simulink model "Sub2_2023"  (R2023b)
settings: Solver=FixedStepDiscrete  StartTime=0.0  StopTime=4.5  FixedStep=7.5e-05  RelTol=1e-3  EnableMultiTasking=on
undefined symbols (not defined in the file or in its folder): D1, D11, Delta
libraries: spsSeriesRLCBranchLib x41, spsLoadFlowBusLib x29, spsDistributedParametersLineLib x19, spsThreePhaseSeriesRLCLoadLib x15, spsThreePhaseTransformerTwoWindingsLib x13, spsThreePhaseParallelRLCLoadLib x11, spsThreePhaseVIMeasurementLib x11, spsSynchronousMachinepuStandardLib x7, spsExcitationSystemLib x7, spsHydraulicTurbineandGovernorLib x7, spsGenericPowerSystemStabilizerLib x7, spsMultiBandPowerSystemStabilizerLib x7
(part 1 of 5)
settings Model: Creator=The MathWorks, Inc.  LastModifiedBy=dilu2
settings SolverCC: AlgebraicLoopSolver=TrustRegion
settings DataIOCC: SaveFormat=StructureWithTime  SaveOutput=off  SignalLogging=off  DSMLogging=off  SaveTime=off  ReturnWorkspaceOutputs=off
settings OptimizationCC: ExpressionDepthLimit=2147483647  LifeSpan=inf
settings DebuggingCC: UnderspecifiedInitializationDetection=Classic  MergeDetectMultiDrivingBlocksExec=none  SolverPrmCheckMsg=warning  FcnCallInpInsideContextMsg=warning  UnconnectedInputMsg=warning  UnconnectedOutputMsg=warning  UnconnectedLineMsg=warning  StateNameClashWarn=warning  SFUnexpectedBacktrackingDiag=warning  SFNoUnconditionalDefaultTransitionDiag=warning  SFExecutionAtInitializationDiag=none  ArithmeticOperatorsInVariantConditions=warning
settings HardwareCC: ProdBitPerPointer=32  ProdBitPerSizeT=32  ProdBitPerPtrDiffT=32  ProdLargestAtomicFloat=None  ProdIntDivRoundTo=Undefined  ProdEndianess=Unspecified  ProdWordSize=32  ProdHWDeviceType=32-bit Generic
settings ModelReferenceCC: EnableRefExpFcnMdlSchedulingChecks=on  PropagateSignalLabelsOutOfModel=off
settings SFSimCC: SimUseLocalCustomCode=off  CustomCodeUndefinedFunction=UseInterfaceOnly
settings RTWCC: RTWUseLocalCustomCode=off
settings CodeAppCC: StateflowObjectComments=on
settings GRTTargetCC: TargetLangStandard=C89/C90 (ANSI)  CombineOutputUpdateFcns=off  GRTInterface=on
settings ConfigComp: CovMetricSettings=dw  CovSaveCumulativeToWorkspaceVar=on  CovSaveSingleToWorkspaceVar=on  CovExternalEMLEnable=off  CovSFcnEnable=off
settings SimscapeCC: SimscapeNormalizeSystem=off

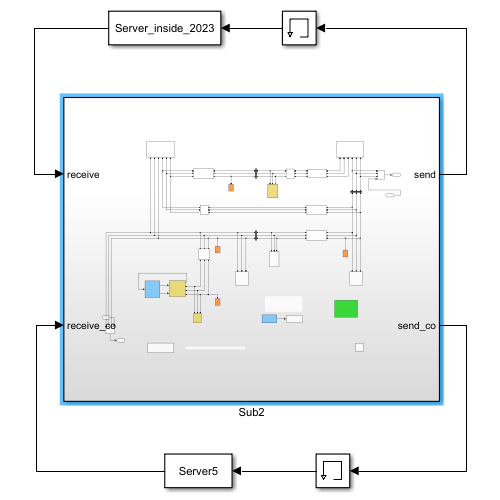
[thumbnail: Simulink's stored preview of the top-level diagram]
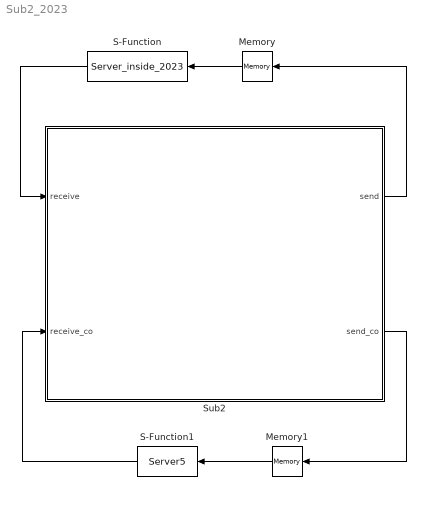
== system Sub2_2023 ==
  Memory : Memory
  Memory1 : Memory
  S-Function : S-Function  FunctionName=Server_inside_2023  SFunctionDeploymentMode=off  EnableBusSupport=off
  S-Function1 : S-Function  FunctionName=Server5  SFunctionDeploymentMode=off  EnableBusSupport=off
  Sub2 : Subsystem
  wires:
  Memory/1 -> S-Function/1
  Sub2/1(send) -> Memory/1
  S-Function/1 -> Sub2/1(receive)
  Memory1/1 -> S-Function1/1
  Sub2/2(send_co) -> Memory1/1
  S-Function1/1 -> Sub2/2(receive_co)

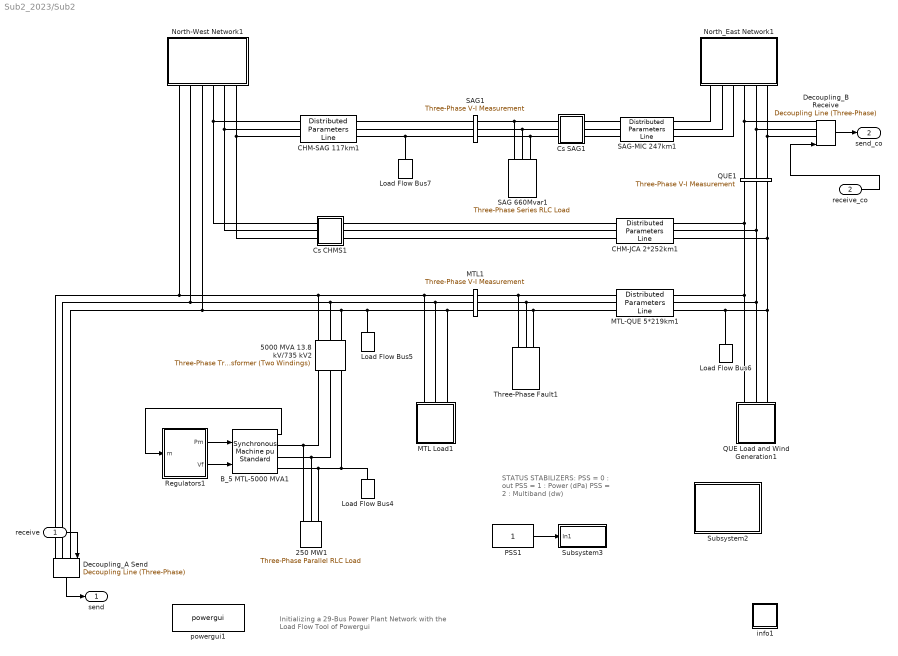
== system Sub2_2023/Sub2 ==
  note: STATUS STABILIZERS:
      | PSS = 0 :  out
      | PSS = 1 :  Power (dPa)
      | PSS = 2 :  Multiband (dw)
  note: Initializing a 29-Bus Power Plant Network with the Load Flow Tool of Powergui
  receive : Inport
  receive_co : Inport  Port=2
  250 MW1 : spsThreePhaseParallelRLCLoadLib/Three-Phase Parallel RLC Load  LConnTagsString=A|B|C  Configuration=Y (grounded)  NominalVoltage=(13800)*1  Vabc=[1e3 1e3 1e3]  Vabcp=[1e3 1e3 1e3]  NominalFrequency=60  UnbalancedPower=off  ActivePower=250000000  InductivePower=0  CapacitivePower=0  Pabc=[10e3 9e3 11e3]  QLabc=[100 90 110]  QCabc=[100 90 110]  Pabcp=[10e3 9e3 11e3]  QLabcp=[100 90 110]  QCabcp=[100 90 110]  Measurements=None  LoadType=constant PQ
  5000 MVA 13.8 kV/735 kV2 : spsThreePhaseTransformerTwoWindingsLib/Three-Phase Transformer (Two Windings)  Winding1Connection=Delta (D1)  Winding2Connection=Yg  CoreType=Three single-phase transformers  SetSaturation=off  Hysteresis=off  DataFile='basic_model'  SetInitialFlux=off  Measurements=None  UNITS=pu  NominalPower=[ 5000e6 60 ]  Winding1="[ 13.8e3 0.002  0.0]"  Winding2=[ 735e3 0.002 0.12]  Rm=500  Lm=500  L0=0.5  Saturation="[ 0,0  ;  0.005,1.2  ;  1.0,1.4 ]"  InitialFluxes=[ 0.8 , -0.8 , 0.7 ]  BreakLoop=off  DiscreteSolver=Trapezoidal iterative  DataType=off  TransfoNumber=0
  B_5 MTL-5000 MVA1 : spsSynchronousMachinepuStandardLib/Synchronous Machine pu Standard  PresetModel=No  MechanicalLoad=Mechanical power Pm  ShowDetailedParameters=on  RotorType=Salient-pole  Units=per unit standard parameters  MeasurementBus=off  NominalParameters="[5000E6  13800   60 ]"  Reactances1=[ 31 32 33 34 35 36 37 ]  Reactances2=[ 1.305, 0.296, 0.252, 0.474, 0.243, 0.18 ]  dAxisTimeConstants=Short-circuit  qAxisTimeConstants=Open-circuit  TimeConstants1=[]  TimeConstants2=[]  TimeConstants3=[]  TimeConstants4=[]  TimeConstants5=[ 1.01, 0.053, 0.1 ]  TimeConstants6=[]  TimeConstants7=[]  TimeConstants8=[]  StatorResistance=2.8544e-3  Mechanical="[ 3.7 0  32]"  PolePairs=32  InitialConditions=[0 -113.876 0.904539 0.904539 0.904539 -42.1129 -162.113 77.8871 1.28555]  SetSaturation=off  Saturation=[0.6404,0.7127,0.8441,0.9214,0.9956,1.082,1.19,1.316,1.457;0.7,0.7698,0.8872,0.9466,0.9969,1.046,1.1,1.151,1.201]  LoadFlowParameters=[1 4000000000 0 0 0]  TsPowergui=0  TsBlock=-1  IterativeModel=Trapezoidal non iterative  IterativeDiscreteModel=Trapezoidal non iterative  BusType=PV  Pref=4500000000  Qref=0  Qmin=-Inf  Qmax=Inf  PLF=0  QLF=0
  CHM-JCA 2*252km1 : spsDistributedParametersLineLib/Distributed Parameters Line  Phases=3  Length=252  Frequency=60  Resistance="[0.01273  0.3864]/2"  Inductance="[0.9337e-3  4.1264e-3]/2"  Capacitance=[12.74e-9 7.751e-9]*2  x1=[-0.0015 2.03650540175105e-08 15714.2625948623 -742648.807936856;-0.001425 2.03802417175712e-08 36703.0761534736 -741907.711972361;-0.00135 2.03791377642309e-08 57662.5498345837 -740573.546334484;-0.001275 2.03617430399732e-08 78575.9289556225 -738647.377534823;-0.0012 2.03280714498745e-08 99426.4956813062 -736130.745323245;-0.001125 2.02781499104887e-08 120197.582387619 -733025.661457033;-0.00105 2.02120183283305e-08 140872.584985655 -729334.608092721;-0.000975 2.01297295679749e-08 161434.976194677 -725060.535801893;-0.0009 2.00313494097978e-08 181868.318753767 -720206.861212544;-0.000825 1.99169564973925e-08 202156.278561524 -714777.464277876;-0.00075 1.97866422747028e-08 222282.637733293 -708776.685174726;-0.000675 1.96405109129245e-08 242231.307565497 -702209.320834094;-0.0006 1.94786792272323e-08 261986.341396696 -695080.621106551;-0.000525 1.93012765833996e-08 281531.947355108 -687396.284565585;-0.00045 1.91084447943856e-08 300852.500982388 -679162.453952253;-0.000375 1.8900338006972e-08 319932.55772358 -670385.711264765;-0.0003 1.86771225785405e-08 338756.86527326 -661073.072496938;-0.000225 1.84389769440892e-08 357310.375767994 -651231.982029715;-0.00015 1.81860914735947e-08 375578.257815372 -640870.306680239;-7.5e-05 1.79186683198327e-08 393545.908349992 -629996.329413249]  x2=[-0.0015 1.37456476437626e-08 -209700.603633318 -700128.672635041;-0.001425 1.37143974011628e-08 -189823.746323575 -705777.196573853;-0.00135 1.36721840791177e-08 -169795.146815422 -710861.533020477;-0.001275 1.36190414223113e-08 -149630.815664857 -715377.617634151;-0.0012 1.35550119121701e-08 -129346.871929678 -719321.840325932;-0.001125 1.34801467329051e-08 -108959.530284152 -722691.048144551;-0.00105 1.33945057305949e-08 -88485.088057253 -725482.547796826;-0.000975 1.32981573653464e-08 -67939.9122048287 -727694.107800648;-0.0009 1.31911786565688e-08 -47340.4262261034 -729323.960268787;-0.000825 1.30736551214049e-08 -26703.0970349858 -730370.802322118;-0.00075 1.29456807063705e-08 -6044.42179666949 -730833.797131121;-0.000675 1.28073577122551e-08 14619.0852599484 -730712.574584829;-0.0006 1.26587967123436e-08 35270.9060434889 -730007.231586691;-0.000525 1.25001164640264e-08 55894.5318044012 -728718.331977109;-0.00045 1.2331443813866e-08 76473.4763318042 -726846.906082708;-0.000375 1.21529135961982e-08 96991.2891323108 -724394.449892715;-0.0003 1.19646685253474e-08 117431.568580302 -721362.923863085;-0.000225 1.1766859081543e-08 137777.975029133 -717754.751349341;-0.00015 1.15596433906279e-08 158014.243872799 -713572.816669385;-7.5e-05 1.13431870976547e-08 178124.198547612 -708820.462797813]  x3=[-0.0015 5.03591321245588e-11 0.894999888084755 -284.908126311335;-0.001425 4.98693784000735e-11 8.94952227197466 -284.768519996507;-0.00135 4.93397598575223e-11 16.9968905446926 -284.401274083898;-0.001275 4.87706998658647e-11 25.0306717631703 -283.806682144272;-0.0012 4.8162653322951e-11 33.0444438456226 -282.985219485328;-0.001125 4.75161062918843e-11 41.0318007052617 -281.937542771746;-0.00105 4.68315756124686e-11 48.9863573712246 -280.664489500261;-0.000975 4.61096084880555e-11 56.9017550926213 -279.167077330181;-0.0009 4.53507820481176e-11 64.7716664216231 -277.446503269882;-0.000825 4.45557028869008e-11 72.5898002715271 -275.504142719944;-0.00075 4.37250065785213e-11 80.3499069457553 -273.341548373669;-0.000675 4.28593571688979e-11 88.0457831337658 -270.960448975891;-0.0006 4.19594466449239e-11 95.6712768698848 -268.362747941035;-0.000525 4.1025994381303e-11 103.220292451094 -265.550521831563;-0.00045 4.00597465654924e-11 110.686795309841 -262.526018697998;-0.000375 3.9061475601212e-11 118.064816837982 -259.291656281869;-0.0003 3.80319794909967e-11 125.348459157995 -255.850020083003;-0.000225 3.69720811982851e-11 132.531899837652 -252.20386129272;-0.00015 3.58826279895553e-11 139.609396544386 -248.356094594567;-7.5e-05 3.47644907570334e-11 146.575291635618 -244.309795834372]  x4=[-0.0015 3.52013720407501e-11 -3172.83341993516 -10043.3125795473;-0.001425 3.62675085587556e-11 -2887.63550825219 -10128.9965094932;-0.00135 3.73046533853308e-11 -2600.12926492622 -10206.5834746083;-0.001275 3.83119774427701e-11 -2310.54451804918 -10276.0114530598;-0.0012 3.92886754916345e-11 -2019.11275723693 -10337.224945184;-0.001125 4.02339667744478e-11 -1726.06694858001 -10390.1750178518;-0.00105 4.11470956398219e-11 -1431.6413484141 -10434.8193435853;-0.000975 4.20273321465133e-11 -1136.07131605911 -10471.1222343937;-0.0009 4.28739726469264e-11 -839.593125676545 -10499.0546703014;-0.000825 4.36863403495994e-11 -542.443777395516 -10518.5943225467;-0.00075 4.44637858602204e-11 -244.860807858507 -10529.7255714304;-0.000675 4.52056877007434e-11 52.9178996618098 -10532.4395188024;-0.0006 4.59114528061887e-11 350.654305422807 -10526.7339951749;-0.000525 4.65805169987294e-11 648.11040349724 -10512.6135614561;-0.00045 4.72123454386872e-11 945.048412031539 -10490.0895053046;-0.000375 4.78064330520745e-11 1241.23096332499 -10459.1798321063;-0.0003 4.83623049343428e-11 1536.42129357782 -10419.9092505811;-0.000225 4.88795167300147e-11 1830.3834321566 -10372.3091530309;-0.00015 4.93576549878944e-11 2122.88239022553 -10316.4175902454;-7.5e-05 4.97963374915741e-11 2413.68434859289 -10252.2792410848]  x5=0.00142516474882927  V1=ones(3,3)  V2=ones(3,3)  I1=ones(3,3)  I2=ones(3,3)  nHarmo=1  Measurements=None  Decoupling=on  VsMag0=[606505.937088319 606505.596193778 606505.952336297]  VrMag0=[596743.737336293 596743.911083344 596743.706580488]  VsAngle0=[3.61218308622256 -116.387796657594 123.612221103652]  VrAngle0=[-14.2738568821762 -134.273869923445 105.726122150017]  IsMag0=[234.023435046343 234.01262310882 234.010085806298]  IrMag0=[8650.90032066054 8650.9061903303 8650.91364627956]  IsAngle0=[2.58186505613148 -117.420380634198 122.583034804858]  IrAngle0=[-15.132183015214 -135.132103549665 104.867823050532]
      settings: AttributesFormatString=\n  LibrarySourceBlock=sps_lib/Power Grid Elements/Distributed Parameters Line
  CHM-SAG 117km1 : spsDistributedParametersLineLib/Distributed Parameters Line  Phases=3  Length=117  Frequency=60  Resistance="[0.01273  0.3864]"  Inductance="[0.9337e-3  4.1264e-3]"  Capacitance=[12.74e-9 7.751e-9]  x1=[-0.000675 1.88816449590376e-08 161384.253868467 -730188.013921256;-0.0006 1.87306893739895e-08 181962.578167366 -725333.731757354;-0.000525 1.85647607624449e-08 202395.444365398 -719899.628906264;-0.00045 1.83839917651972e-08 222666.51874196 -713890.04930666;-0.000375 1.81885268862169e-08 242759.59691035 -707309.796924525;-0.0003 1.79785223771376e-08 262658.616771318 -700164.13191293;-0.000225 1.77541461123506e-08 282347.671352849 -692458.766407155;-0.00015 1.75155774548089e-08 301811.021525966 -684199.859958489;-7.5e-05 1.72630071126472e-08 321033.108586338 -675394.01461038]  x2=[-0.000675 1.29951667225312e-08 211241.020698706 -709610.354234887;-0.0006 1.28653399577539e-08 231217.678579182 -703354.834381639;-0.000525 1.27252288370607e-08 251009.504585151 -696537.063435476;-0.00045 1.25749453631376e-08 270600.677433729 -689162.491418178;-0.000375 1.24146096702944e-08 289975.536241096 -681237.013449779;-0.0003 1.22443499284306e-08 309118.593041565 -672766.965036105;-0.000225 1.20643022405789e-08 328014.545168431 -663759.11700426;-0.00015 1.1874610534106e-08 346648.28748668 -654220.670090137;-7.5e-05 1.16754264456599e-08 365004.924467808 -644159.249182257]  x3=[-0.000675 1.4879769943779e-11 931.801693491408 -3923.77003572373;-0.0006 1.3949741165808e-11 1042.35686429537 -3895.8590867222;-0.000525 1.30085611781872e-11 1152.0787909706 -3864.83384757538;-0.00045 1.20569823457982e-11 1260.87976348774 -3830.71911938476;-0.000375 1.10957653461999e-11 1368.67280801404 -3793.54217294206;-0.0003 1.01256785615549e-11 1475.37175643902 -3753.33272692946;-0.000225 9.1474974643958e-12 1580.89131525584 -3710.12292416287;-0.00015 8.16200399772507e-12 1685.1471337437 -3663.94730589748;-7.5e-05 7.16998594994142e-12 1788.05587139646 -3614.84278421604]  x4=[-0.000675 2.80106439104315e-11 34.742941592912 -1477.3234716757;-0.0006 2.86931941198518e-11 76.4934319413538 -1475.75088744286;-0.000525 2.93528074289132e-11 118.182774610691 -1472.99861053035;-0.00045 2.99889565528289e-11 159.777643778261 -1469.06884106622;-0.000375 3.06011329637228e-11 201.244789142074 -1463.96472044805;-0.0003 3.11888472971385e-11 242.551062500596 -1457.69032883176;-0.000225 3.17516297432302e-11 283.663444250911 -1450.25068187001;-0.00015 3.22890304223214e-11 324.549069784088 -1441.65172670275;-7.5e-05 3.28006197445318e-11 365.175255756646 -1431.90033720318]  x5=0.000661683633385019  V1=ones(3,3)  V2=ones(3,3)  I1=ones(3,3)  I2=ones(3,3)  nHarmo=1  Measurements=None  Decoupling=on  VsMag0=[610584.183721663 610584.009535694 610584.1444302]  VrMag0=[604521.569069069 604521.776249751 604521.56500341]  VsAngle0=[-2.95698942545747 -122.956984245958 117.043027319652]  VrAngle0=[1.15752648645546 -118.842485295532 121.157503589909]  IsMag0=[3301.9247358785 3301.92030404064 3301.91445622829]  IrMag0=[1209.87683704244 1209.87940955581 1209.8866532228]  IsAngle0=[-2.06102029189332 -122.061181862038 117.938965522642]  IrAngle0=[-14.0730509971595 -134.072584557011 105.927076719818]
      settings: AttributesFormatString=\n  LibrarySourceBlock=sps_lib/Power Grid Elements/Distributed Parameters Line
  Cs CHMS1 : Subsystem  mask{Xc=33/2}
      mask prompts: Xc "Condensator Reactance at  60Hz  (ohm):"
      mask help: Series Compensation
      mask init:
      | Cs=1/Xc/(2*pi*60);
      mask Display: disp('Cs')
  Cs SAG1 : Subsystem  mask{Xc=22}
      mask prompts: Xc "Condensator Reactance at  60Hz  (ohm):"
      mask help: Series Compensation
      mask init:
      | Cs=1/Xc/(2*pi*60);
      mask Display: disp('Cs')
  Decoupling_A Send : spsDecouplingLineThreePhaseLib/Decoupling Line (Three-Phase)  Length=252  Frequency=60  Resistance="[0.01273  0.3864]/2"  Inductance="[0.9337e-3  4.1264e-3]/2"  Capacitance=[12.74e-9 7.751e-9]*2  VsMag0=[520613.013364061 520613.032750521 520613.042981028]  VsAngle0=[95.9069967092237 -144.093005822691 -24.0930027089943]  IhsMag0=[3886.83215054636 3886.8322952802 3886.83237166569]  IhsAngle0=[86.4922430479772 -153.50775948401 -33.507756370339]  ShowPorts=on  ConnectorID=T42_4042_2844522148740_S
      settings: LibrarySourceBlock=|
      | sps_lib/Power Grid Elements/Decoupling Line
      | (Three-Phase)
  Decoupling_B Receive : spsDecouplingLineThreePhaseLib/Decoupling Line (Three-Phase)  Length=252  Frequency=60  Resistance="[0.01273  0.3864]/2"  Inductance="[0.9337e-3  4.1264e-3]/2"  Capacitance=[12.74e-9 7.751e-9]*2  VsMag0=[539326.065002421 539326.156042167 539326.020709089]  VsAngle0=[103.825331452963 -136.174657529596 -16.1746546623901]  IhsMag0=[3629.74540446448 3629.74477875113 3629.75000907221]  IhsAngle0=[47.3040516013859 167.303961970595 -72.6960017676645]  ShowPorts=on  ConnectorID=T42_4043_2846767750151_R
      settings: LibrarySourceBlock=|
      | sps_lib/Power Grid Elements/Decoupling Line
      | (Three-Phase)
  Load Flow Bus4 : spsLoadFlowBusLib/Load Flow Bus  LConnTagsString=a  Phases=single  Connectors=on one side  ID=MTL_13.8  Vbase=13.8e3  Vref=1  Vangle=0  VLF=1  VLFb=1  VLFc=1  angleLF=-47.86  angleLFb=0  angleLFc=0
      settings: AttributesFormatString=%<ID>\n%<Vbase>V\n%<VLF>pu\n%<angleLF>deg.
  Load Flow Bus5 : spsLoadFlowBusLib/Load Flow Bus  LConnTagsString=a  Phases=single  Connectors=on one side  ID=MTL7  Vbase=735e3  Vref=1  Vangle=0  VLF=1.013  VLFb=1  VLFc=1  angleLF=-23.64  angleLFb=0  angleLFc=0
      settings: AttributesFormatString=%<ID>\n%<Vbase>V\n%<VLF>pu\n%<angleLF>deg.
  Load Flow Bus6 : spsLoadFlowBusLib/Load Flow Bus  LConnTagsString=a  Phases=single  Connectors=on one side  ID=QUE7  Vbase=735e3  Vref=1  Vangle=0  VLF=1.023  VLFb=1  VLFc=1  angleLF=-14.99  angleLFb=0  angleLFc=0
      settings: AttributesFormatString=%<ID>\n%<Vbase>V\n%<VLF>pu\n%<angleLF>deg.
  Load Flow Bus7 : spsLoadFlowBusLib/Load Flow Bus  LConnTagsString=a  Phases=single  Connectors=on one side  ID=SAG7  Vbase=735e3  Vref=1  Vangle=0  VLF=1.036  VLFb=1  VLFc=1  angleLF=-0.1653  angleLFb=0  angleLFc=0
      settings: AttributesFormatString=%<ID>\n%<Vbase>V\n%<VLF>pu\n%<angleLF>deg.
  MTL Load1 : Subsystem
  MTL-QUE 5*219km1 : spsDistributedParametersLineLib/Distributed Parameters Line  Phases=3  Length=219  Frequency=60  Resistance="[0.01273  0.3864]/5"  Inductance="[0.9337e-3  4.1264e-3]/5"  Capacitance=[12.74e-9 7.751e-9]*5  x1=[-0.001275 8.55247461198174e-08 0 0;-0.0012 8.55018995029049e-08 0 0;-0.001125 8.54107039757528e-08 0 0;-0.00105 8.525123243867e-08 0 0;-0.000975 8.50236123707633e-08 0 0;-0.0009 8.47280257280323e-08 0 0;-0.000825 8.43647087979166e-08 -143097.879675135 -713663.77653516;-0.00075 8.39339520104112e-08 -122864.99863668 -717423.987747288;-0.000675 8.34360997059012e-08 -102533.901198211 -720610.701200567;-0.0006 8.28715498599015e-08 -82120.8397279466 -723221.369485019;-0.000525 8.22407537649209e-08 -61642.1321148943 -725253.905672363;-0.00045 8.15442156697064e-08 -41114.1487245856 -726706.684984269;-0.000375 8.07824923761539e-08 -20553.2993128541 -727578.546091184;-0.0003 7.99561927942095e-08 23.9800918721885 -727868.792040679;-0.000225 7.90659774551161e-08 20601.2403272799 -727577.190814582;-0.00015 7.81125579833952e-08 41162.0322463795 -726703.975514453;-7.5e-05 7.70966965279846e-08 61689.9198667016 -725249.84417524]  x2=[-0.001275 1.36190414223113e-08 0 0;-0.0012 1.35550119121701e-08 0 0;-0.001125 1.34801467329051e-08 0 0;-0.00105 1.33945057305949e-08 0 0;-0.000975 1.32981573653464e-08 0 0;-0.0009 1.31911786565688e-08 0 0;-0.000825 1.30736551214049e-08 -26703.0970349858 -730370.802322118;-0.00075 1.29456807063705e-08 -6044.42179666949 -730833.797131121;-0.000675 1.28073577122551e-08 14619.0852599484 -730712.574584829;-0.0006 1.26587967123436e-08 35270.9060434889 -730007.231586691;-0.000525 1.25001164640264e-08 55894.5318044012 -728718.331977109;-0.00045 1.2331443813866e-08 76473.4763318042 -726846.906082708;-0.000375 1.21529135961982e-08 96991.2891323108 -724394.449892715;-0.0003 1.19646685253474e-08 117431.568580302 -721362.923863085;-0.000225 1.1766859081543e-08 137777.975029133 -717754.751349341;-0.00015 1.15596433906279e-08 158014.243872799 -713572.816669385;-7.5e-05 1.13431870976547e-08 178124.198547612 -708820.462797813]  x3=[-0.001275 3.39337734391403e-10 0 0;-0.0012 3.15137628564504e-10 0 0;-0.001125 2.90685606539098e-10 0 0;-0.00105 2.66001214887464e-10 0 0;-0.000975 2.41104185934603e-10 0 0;-0.0009 2.16014421984524e-10 0 0;-0.000825 1.90751979410642e-10 -5323.24056616418 -20344.1866352304;-0.00075 1.65337052623023e-10 -4745.97060123289 -20486.5462812054;-0.000675 1.39789957925278e-10 -4164.90678001876 -20612.5292955377;-0.0006 1.14131117274026e-10 -3580.51359604989 -20722.0349693336;-0.000525 8.83810419538894e-11 -2993.25820429603 -20814.9757654327;-0.00045 6.25603161810904e-11 -2403.61004773205 -20891.2773883847;-0.000375 3.66895806487412e-11 -1812.04048207238 -20950.8788438397;-0.0003 1.07895160269909e-11 -1219.02239897648 -20993.7324873061;-0.000225 -1.51191735687863e-11 -625.029848026517 -21019.8040622371;-0.00015 -4.10157771285438e-11 -30.5376577793149 -21029.0727274145;-7.5e-05 -6.68795933036271e-11 563.978943804274 -21021.5310736092]  x4=[-0.001275 2.90453714362749e-10 0 0;-0.0012 3.18276510024189e-10 0 0;-0.001125 3.4584488031331e-10 0 0;-0.00105 3.73136787496712e-10 0 0;-0.000975 4.00130414841374e-10 0 0;-0.0009 4.26804184054612e-10 0 0;-0.000825 4.5313677253344e-10 -1592.00824148655 -5672.40977476736;-0.00075 4.7910713040953e-10 -1431.01007071885 -5715.14957069222;-0.000675 5.04694497376155e-10 -1268.8679723958 -5753.32076349499;-0.0006 5.29878419283663e-10 -1105.71156042995 -5786.89283970819;-0.000525 5.54638764490207e-10 -941.671259560641 -5815.83896232775;-0.00045 5.78955739954675e-10 -776.878201094496 -5840.13599226614;-0.000375 6.02809907058943e-10 -611.464118081032 -5859.7645068494;-0.0003 6.2618219714681e-10 -445.561240007288 -5874.70881534328;-0.000225 6.49053926767186e-10 -279.302187095599 -5884.95697149624;-0.00015 6.71406812609362e-10 -112.819864289011 -5890.50078308904;-7.5e-05 6.93222986118407e-10 53.752644990887 -5891.33581848353]  x5=0.00123853603172068  V1=ones(3,3)  V2=ones(3,3)  I1=ones(3,3)  I2=ones(3,3)  nHarmo=1  Measurements=None  Decoupling=on  VsMag0=[594302.518281082 594302.525591459 594302.380387508]  VrMag0=[596743.737336293 596743.911083344 596743.706580488]  VsAngle0=[-23.5181046800034 -143.518120437634 96.481886830827]  VrAngle0=[-14.2738568821762 -134.273869923445 105.726122150017]  IsMag0=[17258.8321886657 17258.8369567339 17258.8217052479]  IrMag0=[4835.28137561885 4835.27973459301 4835.28879562026]  IsAngle0=[-26.8431826212219 -146.843231946898 93.1567790076113]  IrAngle0=[-27.8572964469064 -147.857183694794 92.1427767692856]
      settings: AttributesFormatString=\n  LibrarySourceBlock=sps_lib/Power Grid Elements/Distributed Parameters Line
  MTL1 : spsThreePhaseVIMeasurementLib/Three-Phase V-I Measurement  VoltageMeasurement=phase-to-ground  SetLabelV=on  LabelV=Vabc_MTL7_1  Vpu=on  VpuLL=off  CurrentMeasurement=no  SetLabelI=off  LabelI=A1  Ipu=off  Pbase=100e6  Vbase=735e3  OutputType=Magnitude  PhasorSimulation=off  PSBequivalent=0
  North-West Network1 : Subsystem
  North_East Network1 : Subsystem
  PSS1 : Constant
  QUE Load and Wind Generation1 : Subsystem
  QUE1 : spsThreePhaseVIMeasurementLib/Three-Phase V-I Measurement  VoltageMeasurement=no  SetLabelV=on  LabelV=Vabc_QUE7  Vpu=on  VpuLL=off  CurrentMeasurement=no  SetLabelI=off  LabelI=A1  Ipu=off  Pbase=100e6  Vbase=735e3  OutputType=Magnitude  PhasorSimulation=off  PSBequivalent=0
  Regulators1 : Subsystem
  SAG 660Mvar1 : spsThreePhaseSeriesRLCLoadLib/Three-Phase Series RLC Load  LConnTagsString=A|B|C  Configuration=Y (grounded)  NominalVoltage=735e3  Vabc=[1e3 1e3 1e3]  Vabcp=[1e3 1e3 1e3]  NominalFrequency=60  UnbalancedPower=off  ActivePower=2200000  InductivePower=660e6  CapacitivePower=0  Pabc=[10e3 9e3 11e3]  QLabc=[100 90 110]  QCabc=[100 90 110]  Pabcp=[10e3 9e3 11e3]  QLabcp=[100 90 110]  QCabcp=[100 90 110]  Measurements=None  LoadType=constant Z
  SAG-MIC 247km1 : spsDistributedParametersLineLib/Distributed Parameters Line  Phases=3  Length=247  Frequency=60  Resistance="[0.01273  0.3864]/1"  Inductance="[0.9337e-3  4.1264e-3]/1"  Capacitance=[12.74e-9 7.751e-9]*1  x1=[-0.001425 1.43932636664465e-08 -23892.3616667482 -729222.08414719;-0.00135 1.43732239636393e-08 -3267.28940137557 -729606.070163733;-0.001275 1.43416945255134e-08 17360.3946851533 -729406.820251135;-0.0012 1.4298700556219e-08 37974.2011377939 -728624.493686727;-0.001125 1.42442764244774e-08 58557.6515950696 -727259.715850394;-0.00105 1.41784656361068e-08 79094.2919616224 -725313.577724657;-0.000975 1.41013207992446e-08 99567.7055613643 -722787.635022557;-0.0009 1.40129035822928e-08 119961.526260717 -719683.906944042;-0.000825 1.3913284664622e-08 140259.451551451 -716004.874561848;-0.00075 1.38025436800707e-08 160445.255582655 -711753.478838172;-0.000675 1.36807691532876e-08 180502.802131442 -706933.118273706;-0.0006 1.3548058428966e-08 200416.05750199 -701547.646190932;-0.000525 1.34045175940287e-08 220169.103342639 -695601.367653831;-0.00045 1.32502613928226e-08 239746.149370777 -689099.036026485;-0.000375 1.30854131353949e-08 259131.545995347 -682045.849173309;-0.0003 1.29101045989203e-08 278309.796826893 -674447.445303955;-0.000225 1.27244759223606e-08 297265.571065139 -666309.898466218;-0.00015 1.25286754944396e-08 315983.715754192 -657639.713690529;-7.5e-05 1.23228598350234e-08 334449.267895583 -648443.821789942]  x2=[-0.001425 4.54303378111499e-09 88893.3544414479 -739233.912944377;-0.00135 4.5056705027986e-09 109756.403307744 -736425.413362135;-0.001275 4.46470546042134e-09 130531.714584565 -733028.226572137;-0.0012 4.42017140081131e-09 151202.680805949 -729045.068233526;-0.001125 4.37210392381436e-09 171752.777917775 -724479.122422133;-0.00105 4.32054145383614e-09 192165.57848684 -719334.039085178;-0.000975 4.26552520912623e-09 212424.764832694 -713613.931123558;-0.0009 4.20709916882887e-09 232514.142071749 -707323.371104057;-0.000825 4.14531003782672e-09 252417.651063218 -700467.387604106;-0.00075 4.08020720940571e-09 272119.381246546 -693051.461192015;-0.000675 4.01184272577075e-09 291603.583360071 -685081.520045889;-0.0006 3.94027123644407e-09 310854.682030743 -676563.935214738;-0.000525 3.86554995457915e-09 329857.288224836 -667505.515525552;-0.00045 3.78773861122544e-09 348596.211549708 -657913.502140431;-0.000375 3.70689940758025e-09 367056.472396768 -647795.562768113;-0.0003 3.62309696526611e-09 385223.313915946 -637159.785534523;-0.000225 3.53639827467318e-09 403082.213812094 -626014.672517248;-0.00015 3.44687264140818e-09 420618.895953885 -614369.132949109;-7.5e-05 3.35459163089256e-09 437819.341785936 -602232.476096253]  x3=[-0.001425 1.48732714466042e-11 -591.222973545599 -3970.47337116351;-0.00135 1.42908317856594e-11 -478.738749484937 -3985.60043687626;-0.001275 1.36969682524421e-11 -365.871828992885 -3997.5414745815;-0.0012 1.30921555723745e-11 -252.712436158763 -4006.28693879639;-0.001125 1.2476877223459e-11 -139.351028869805 -4011.82983853066;-0.00105 1.18516250497937e-11 -25.8782265005118 -4014.16574287506;-0.000975 1.12168988683996e-11 87.6152625270965 -4013.2927845434;-0.0009 1.05732060696743e-11 201.038713254399 -4009.21166136522;-0.000825 9.92106121179248e-12 314.301456710321 -4001.92563572793;-0.00075 9.26098560937524e-12 427.312952390723 -3991.44053196896;-0.000675 8.5935069167597e-12 539.98286063509 -3977.76473171983;-0.0006 7.91915870619997e-12 652.221114842681 -3960.90916720599;-0.000525 7.23848004133769e-12 763.937993470385 -3940.88731250784;-0.00045 6.55201504628282e-12 875.044191754751 -3917.71517278966;-0.000375 5.86031247064915e-12 985.450893100854 -3891.41127150541;-0.0003 5.16392525089223e-12 1095.06984008092 -3861.9966355913;-0.000225 4.46341006830045e-12 1203.81340498595 -3829.49477865724;-0.00015 3.75932690399254e-12 1311.594659874 -3793.93168219035;-7.5e-05 3.0522385912772e-12 1418.32744605901 -3755.33577478582]  x4=[-0.001425 1.10984325063843e-11 -44.2696955263769 -1445.03567528016;-0.00135 1.17732015549195e-11 -3.40032222028924 -1445.70991618406;-0.001275 1.24385592862677e-11 37.4717692513545 -1445.22847870107;-0.0012 1.30939738236389e-11 78.3139063639962 -1443.59174768495;-0.001125 1.37389212386799e-11 119.093440538133 -1440.80103151342;-0.00105 1.43728859702953e-11 159.777773238095 -1436.85856104229;-0.000975 1.49953612367786e-11 200.334382030812 -1431.76748782214;-0.0009 1.56058494409259e-11 240.730846583753 -1425.531881579;-0.000825 1.62038625678076e-11 280.93487458124 -1418.1567269611;-0.00075 1.678892257488e-11 320.914327538434 -1409.64791955419;-0.000675 1.73605617741252e-11 360.637246492348 -1400.01226116872;-0.0006 1.79183232059137e-11 400.071877549351 -1389.25745440259;-0.000525 1.84617610042909e-11 439.186697268746 -1377.39209648375;-0.00045 1.89904407533957e-11 477.950437862126 -1364.42567239779;-0.000375 1.95039398347257e-11 516.332112188366 -1350.36854730573;-0.0003 2.00018477649721e-11 554.30103852427 -1335.23195825828;-0.000225 2.04837665241537e-11 591.826865091067 -1319.02800521314;-0.00015 2.09493108737881e-11 628.879594317164 -1301.76964136243;-7.5e-05 2.13981086648452e-11 665.429606817746 -1283.47066277817]  x5=0.00139688767047948  V1=ones(3,3)  V2=ones(3,3)  I1=ones(3,3)  I2=ones(3,3)  nHarmo=1  Measurements=None  Decoupling=on  VsMag0=[595726.85858568 595726.856922657 595726.834929878]  VrMag0=[607930.231676026 607930.976808573 607930.152147035]  VsAngle0=[-1.09657636565014 -121.096578900444 118.903422505471]  VrAngle0=[7.63692875074031 -112.363120449614 127.636843332411]  IsMag0=[3296.72064632848 3296.71771518531 3296.71033953585]  IrMag0=[1187.28543067541 1187.2922723967 1187.29553954548]  IsAngle0=[-7.68926033427173 -127.689437762269 112.310695069129]  IrAngle0=[-0.975042579726905 -120.974669903291 119.024857828972]
      settings: AttributesFormatString=\n  LibrarySourceBlock=sps_lib/Power Grid Elements/Distributed Parameters Line
  SAG1 : spsThreePhaseVIMeasurementLib/Three-Phase V-I Measurement  VoltageMeasurement=no  SetLabelV=on  LabelV=Vabc_SAG7  Vpu=on  VpuLL=off  CurrentMeasurement=no  SetLabelI=off  LabelI=Iabc_SAG7  Ipu=off  Pbase=100e6  Vbase=735e3  OutputType=Magnitude  PhasorSimulation=off  PSBequivalent=0
  Subsystem2 : Subsystem
      mask Display: disp('Display\nWaveforms')
  Subsystem3 : Subsystem
      mask Display: disp('PSS_select')
  Three-Phase Fault1 : spsThreePhaseFaultLib/Three-Phase Fault  InitialStates=0  FaultA=on  FaultB=on  FaultC=on  GroundFault=on  SwitchTimes=[0.2 0.3]  External=off  SwitchStatus=NaN  FaultResistance=0.001  GroundResistance=0.001  SnubberResistance=1e6  SnubberCapacitance=inf  Measurements=None
  info1 : Subsystem
      settings: OpenFcn="showExample(\"simscapeelectricalsps/LoadFlow29BusNetworkExample\")"
      mask Display: disp('?')
  powergui1 : spspowerguiLib/powergui  Priority=1  SimulationMode=Discrete  SampleTime=75e-6  frequency=60  Iterations=50  frequencyindice=60  Pbase=1e+008  ErrMax=0.0001  UnitsV=kV  UnitsW=MW  buscounter=0  FunctionMessages=off  echomessages=off  EnableUseOfTLC=off  CurrentSourceSwitches=off  DisableSnubberDevices=off  DisableRonSwitches=off  DisableVfSwitches=off  DisplayEquations=off  AutomaticDiscreteSolvers=off  SolverType=Tustin/Backward Euler (TBE)  Interpol=off  ExternalGateDelay=off  methode=off  Ts=100  x0status=blocks  SPID=off  SwTol=0  HookPort=off  NonlinearTolerance=1e-4  nMaxIteration=100  ContinueOnMaxIteration=off  RestoreLinks=warning  ResistiveCurrentMeasurement=off  Frange=[0:2:500]  Ylog=off  Xlog=on  ShowGrid=off  save=off  variable=ZData  structure=0  ZoomFFT=off  StartTime=0.0  cycles=1  DisplayStyle=1  fundamental=60  FreqAxis=off  MaxFrequency=1000  frequencyindicesteady=1  RmsSteady=1  display=off
  send : Outport
  send_co : Outport  Port=2
  wires:
  Regulators1/2(Vf) -> B_5 MTL-5000 MVA1/2
  receive/1 -> Decoupling_A Send/1
  Regulators1/1(Pm) -> B_5 MTL-5000 MVA1/1
  B_5 MTL-5000 MVA1/1 -> Regulators1/1(m)
  PSS1/1 -> Subsystem3/1(In1)
  Decoupling_A Send/1 -> send/1
  receive_co/1 -> Decoupling_B Receive/1
  Decoupling_B Receive/1 -> send_co/1
  connections:
  MTL-QUE 5*219km1/LConn3 -- MTL1/RConn3 -- Three-Phase Fault1/LConn3
  MTL Load1/LConn1 -- MTL1/LConn1 -- Decoupling_A Send/LConn3 -- North-West Network1/RConn1 -- 5000 MVA 13.8 kV/735 kV2/RConn1
  Load Flow Bus6/LConn1 -- QUE1/LConn3 -- CHM-JCA 2*252km1/RConn3 -- QUE Load and Wind Generation1/LConn3 -- MTL-QUE 5*219km1/RConn3
  MTL-QUE 5*219km1/LConn1 -- MTL1/RConn1 -- Three-Phase Fault1/LConn1
  250 MW1/LConn1 -- 5000 MVA 13.8 kV/735 kV2/LConn1 -- B_5 MTL-5000 MVA1/RConn1
  5000 MVA 13.8 kV/735 kV2/RConn3 -- Decoupling_A Send/LConn1 -- North-West Network1/RConn3 -- MTL1/LConn3 -- MTL Load1/LConn3 -- Load Flow Bus5/LConn1
  MTL-QUE 5*219km1/RConn2 -- QUE1/LConn2 -- CHM-JCA 2*252km1/RConn2 -- QUE Load and Wind Generation1/LConn2
  QUE1/RConn2 -- Decoupling_B Receive/LConn2 -- North_East Network1/LConn5
  CHM-SAG 117km1/LConn1 -- North-West Network1/RConn4 -- Cs CHMS1/LConn1
  SAG1/RConn2 -- SAG 660Mvar1/LConn2 -- Cs SAG1/LConn2
  QUE1/RConn1 -- Decoupling_B Receive/LConn3 -- North_East Network1/LConn4
  5000 MVA 13.8 kV/735 kV2/RConn2 -- Decoupling_A Send/LConn2 -- North-West Network1/RConn2 -- MTL1/LConn2 -- MTL Load1/LConn2
  SAG1/RConn1 -- SAG 660Mvar1/LConn1 -- Cs SAG1/LConn1
  SAG1/RConn3 -- SAG 660Mvar1/LConn3 -- Cs SAG1/LConn3
  SAG-MIC 247km1/RConn2 -- North_East Network1/LConn2
  250 MW1/LConn2 -- 5000 MVA 13.8 kV/735 kV2/LConn2 -- B_5 MTL-5000 MVA1/RConn2
  CHM-SAG 117km1/RConn3 -- SAG1/LConn3 -- Load Flow Bus7/LConn1
  CHM-SAG 117km1/LConn3 -- North-West Network1/RConn6 -- Cs CHMS1/LConn3
  CHM-SAG 117km1/LConn2 -- North-West Network1/RConn5 -- Cs CHMS1/LConn2
  Cs SAG1/RConn3 -- SAG-MIC 247km1/LConn3
  Cs SAG1/RConn1 -- SAG-MIC 247km1/LConn1
  MTL-QUE 5*219km1/LConn2 -- MTL1/RConn2 -- Three-Phase Fault1/LConn2
  MTL-QUE 5*219km1/RConn1 -- QUE1/LConn1 -- CHM-JCA 2*252km1/RConn1 -- QUE Load and Wind Generation1/LConn1
  Cs CHMS1/RConn1 -- CHM-JCA 2*252km1/LConn1
  SAG-MIC 247km1/RConn3 -- North_East Network1/LConn3
  SAG1/LConn1 -- CHM-SAG 117km1/RConn1
  SAG1/LConn2 -- CHM-SAG 117km1/RConn2
  QUE1/RConn3 -- Decoupling_B Receive/LConn1 -- North_East Network1/LConn6
  Cs SAG1/RConn2 -- SAG-MIC 247km1/LConn2
  Cs CHMS1/RConn3 -- CHM-JCA 2*252km1/LConn3
  Cs CHMS1/RConn2 -- CHM-JCA 2*252km1/LConn2
  SAG-MIC 247km1/RConn1 -- North_East Network1/LConn1
  5000 MVA 13.8 kV/735 kV2/LConn3 -- 250 MW1/LConn3 -- B_5 MTL-5000 MVA1/RConn3 -- Load Flow Bus4/LConn1

== system Sub2_2023/Sub2/Cs CHMS1 ==
  note: B
  Ca : spsSeriesRLCBranchLib/Series RLC Branch  LConnTagsString=__new0  RConnTagsString=__new0  BranchType=C  Resistance=1.0  Inductance=1.0  SetiL0=off  InitialCurrent=0  Capacitance=Cs  Setx0=off  InitialVoltage=0  Measurements=None
  Cb : spsSeriesRLCBranchLib/Series RLC Branch  LConnTagsString=__new0  RConnTagsString=__new0  BranchType=C  Resistance=1.0  Inductance=1.0  SetiL0=off  InitialCurrent=0  Capacitance=Cs  Setx0=off  InitialVoltage=0  Measurements=None
  Cc : spsSeriesRLCBranchLib/Series RLC Branch  LConnTagsString=__new0  RConnTagsString=__new0  BranchType=C  Resistance=1.0  Inductance=1.0  SetiL0=off  InitialCurrent=0  Capacitance=Cs  Setx0=off  InitialVoltage=0  Measurements=None
  A : PMIOPort  Side=Left
  B : PMIOPort  Port=2  Side=Left
  C : PMIOPort  Port=3  Side=Left
  "A " : PMIOPort  Port=4  Side=Right
  "B " : PMIOPort  Port=5  Side=Right
  "C " : PMIOPort  Port=6  Side=Right
  connections:
  Cc/RConn1 -- "C "/RConn1
  C/RConn1 -- Cc/LConn1
  Cb/RConn1 -- "B "/RConn1
  B/RConn1 -- Cb/LConn1
  Ca/RConn1 -- "A "/RConn1
  A/RConn1 -- Ca/LConn1

== system Sub2_2023/Sub2/Cs SAG1 ==
  note: B
  Ca : spsSeriesRLCBranchLib/Series RLC Branch  LConnTagsString=__new0  RConnTagsString=__new0  BranchType=C  Resistance=1.0  Inductance=1.0  SetiL0=off  InitialCurrent=0  Capacitance=Cs  Setx0=off  InitialVoltage=0  Measurements=None
  Cb : spsSeriesRLCBranchLib/Series RLC Branch  LConnTagsString=__new0  RConnTagsString=__new0  BranchType=C  Resistance=1.0  Inductance=1.0  SetiL0=off  InitialCurrent=0  Capacitance=Cs  Setx0=off  InitialVoltage=0  Measurements=None
  Cc : spsSeriesRLCBranchLib/Series RLC Branch  LConnTagsString=__new0  RConnTagsString=__new0  BranchType=C  Resistance=1.0  Inductance=1.0  SetiL0=off  InitialCurrent=0  Capacitance=Cs  Setx0=off  InitialVoltage=0  Measurements=None
  A : PMIOPort  Side=Left
  B : PMIOPort  Port=2  Side=Left
  C : PMIOPort  Port=3  Side=Left
  "A " : PMIOPort  Port=4  Side=Right
  "B " : PMIOPort  Port=5  Side=Right
  "C " : PMIOPort  Port=6  Side=Right
  connections:
  A/RConn1 -- Ca/LConn1
  Ca/RConn1 -- "A "/RConn1
  B/RConn1 -- Cb/LConn1
  Cb/RConn1 -- "B "/RConn1
  C/RConn1 -- Cc/LConn1
  Cc/RConn1 -- "C "/RConn1

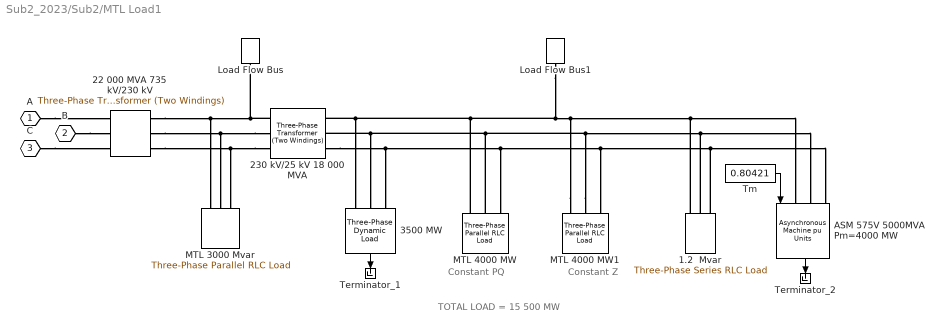
== system Sub2_2023/Sub2/MTL Load1 ==
  note: Constant PQ
  note: Constant Z
  note: TOTAL LOAD = 15 500 MW
  1.2  Mvar : spsThreePhaseSeriesRLCLoadLib/Three-Phase Series RLC Load  LConnTagsString=A|B|C  Configuration=Y (grounded)  NominalVoltage=25e3  Vabc=[1e3 1e3 1e3]  Vabcp=[1e3 1e3 1e3]  NominalFrequency=60  UnbalancedPower=off  ActivePower=2000e6/50  InductivePower=0  CapacitivePower=2000e6  Pabc=[10e3 9e3 11e3]  QLabc=[100 90 110]  QCabc=[100 90 110]  Pabcp=[10e3 9e3 11e3]  QLabcp=[100 90 110]  QCabcp=[100 90 110]  Measurements=None  LoadType=constant Z
  22 000 MVA 735 kV/230 kV : spsThreePhaseTransformerTwoWindingsLib/Three-Phase Transformer (Two Windings)  Winding1Connection=Yg  Winding2Connection=Delta (D1)  CoreType=Three single-phase transformers  SetSaturation=off  Hysteresis=off  DataFile='basic_model'  SetInitialFlux=off  Measurements=None  UNITS=pu  NominalPower=[ 22000e6 60 ]  Winding1="[ 735e3 0.002  0.12]"  Winding2=[230e3 0.002 0]  Rm=500  Lm=500  L0=0.5  Saturation="[ 0,0  ;  0.005,1.2  ;  1.0,1.4 ]"  InitialFluxes=[ 0.8 , -0.8 , 0.7 ]  BreakLoop=off  DiscreteSolver=Trapezoidal iterative  DataType=off  TransfoNumber=0
  230 kV/25 kV 18 000 MVA : spsThreePhaseTransformerTwoWindingsLib/Three-Phase Transformer (Two Windings)  Winding1Connection=Yg  Winding2Connection=Delta (D1)  CoreType=Three single-phase transformers  SetSaturation=off  Hysteresis=off  DataFile='basic_model'  SetInitialFlux=off  Measurements=None  UNITS=pu  NominalPower=[18000e6 60 ]  Winding1="[ 230e3  0.08/30   0.08 ]"  Winding2="[ 25e3  0.08/30  0.08]"  Rm=500  Lm=500  L0=0.5  Saturation="[ 0,0  ;  0.005,1.2  ;  1.0,1.4 ]"  InitialFluxes=[ 0.8 , -0.8 , 0.7 ]  BreakLoop=off  DiscreteSolver=Trapezoidal iterative  DataType=off  TransfoNumber=0
  3500 MW : spsThreePhaseDynamicLoadLib/Three-Phase Dynamic Load  NominalVoltage=[ 25e3 60 ]  ActiveReactivePowers=[3.5e+09 4.44089e-08]  PositiveSequence=[0.991615 -96.3945]  ExternalControl=off  NpNq="[1.5  2.5]"  TimeConstants="[0  0  0  0]"  MinimumVoltage=0.7  Tfilter=1e-4  LoadFlowParameters=[4,0,0,0,0]
      settings: LibrarySourceBlock=|
      | sps_lib/Passives/Three-Phase
      | Dynamic Load
  ASM 575V 5000MVA Pm=4000 MW : spsAsynchronousMachinepuUnitsLib/Asynchronous Machine pu Units  RotorType=Squirrel-cage  PresetModel=No  MechanicalLoad=Torque Tm  ShowDetailedParameters=on  ReferenceFrame=Rotor  Units=pu  MeasurementBus=off  NominalParameters="[5000e6 25e3  60]"  VoltageRatio=1  Stator=[0.01117 0.04832]  Rotor=[0.006 0.04832]  Cage1=[0.01909 0.0397]  Cage2=[0.01909 0.0397]  Lm=2.424  Mechanical="[1  0   2]"  PolePairs=2  InitialConditions=[0.00523668 0 0.941796 0.941796 0.941796 -125.733 -245.733 -5.73298]  SimulateSaturation=off  Saturation="[0.212,0.4201,0.8125,1.0979,1.4799,2.2457,3.2586,4.5763,6.4763 ;   0.5,0.7,0.9,1,1.1,1.2 ,1.3,1.4,1.5]"  LoadFlowParameters=0  TsPowergui=0  TsBlock=-1  IterativeModel=Trapezoidal non iterative  IterativeDiscreteModel=Trapezoidal non iterative  Pmec=4000000000
      settings: LibrarySourceBlock=|
      | sps_lib/Electrical Machines/Asynchronous Machine
      | pu Units
  Load Flow Bus : spsLoadFlowBusLib/Load Flow Bus  LConnTagsString=a  Phases=single  Connectors=on one side  ID=MTL2  Vbase=230e3  Vref=1  Vangle=0  VLF=1.009  VLFb=1  VLFc=1  angleLF=-58.45  angleLFb=0  angleLFc=0
      settings: AttributesFormatString=%<ID>\n%<Vbase>V\n%<VLF>pu\n%<angleLF>deg.
  Load Flow Bus1 : spsLoadFlowBusLib/Load Flow Bus  LConnTagsString=a  Phases=single  Connectors=on one side  ID=MTL_25  Vbase=25e3  Vref=1  Vangle=0  VLF=0.9916  VLFb=1  VLFc=1  angleLF=-96.39  angleLFb=0  angleLFc=0
      settings: AttributesFormatString=%<ID>\n%<Vbase>V\n%<VLF>pu\n%<angleLF>deg.
  MTL 3000 Mvar : spsThreePhaseParallelRLCLoadLib/Three-Phase Parallel RLC Load  LConnTagsString=A|B|C  Configuration=Y (grounded)  NominalVoltage=230e3  Vabc=[1e3 1e3 1e3]  Vabcp=[1e3 1e3 1e3]  NominalFrequency=60  UnbalancedPower=off  ActivePower=0  InductivePower=0  CapacitivePower=3000e6  Pabc=[10e3 9e3 11e3]  QLabc=[100 90 110]  QCabc=[100 90 110]  Pabcp=[10e3 9e3 11e3]  QLabcp=[100 90 110]  QCabcp=[100 90 110]  Measurements=None  LoadType=constant Z
  MTL 4000 MW : spsThreePhaseParallelRLCLoadLib/Three-Phase Parallel RLC Load  LConnTagsString=A|B|C  Configuration=Y (grounded)  NominalVoltage=(25000)*0.991615  Vabc=[1e3 1e3 1e3]  Vabcp=[1e3 1e3 1e3]  NominalFrequency=60  UnbalancedPower=off  ActivePower=4000000000  InductivePower=0  CapacitivePower=0  Pabc=[10e3 9e3 11e3]  QLabc=[100 90 110]  QCabc=[100 90 110]  Pabcp=[10e3 9e3 11e3]  QLabcp=[100 90 110]  QCabcp=[100 90 110]  Measurements=None  LoadType=constant PQ
  MTL 4000 MW1 : spsThreePhaseParallelRLCLoadLib/Three-Phase Parallel RLC Load  LConnTagsString=A|B|C  Configuration=Y (grounded)  NominalVoltage=25e3  Vabc=[1e3 1e3 1e3]  Vabcp=[1e3 1e3 1e3]  NominalFrequency=60  UnbalancedPower=off  ActivePower=4000000000  InductivePower=0  CapacitivePower=0  Pabc=[10e3 9e3 11e3]  QLabc=[100 90 110]  QCabc=[100 90 110]  Pabcp=[10e3 9e3 11e3]  QLabcp=[100 90 110]  QCabcp=[100 90 110]  Measurements=None  LoadType=constant Z
  Terminator_1 : Terminator
  Terminator_2 : Terminator
  Tm : Constant  Value=0.80421
  A : PMIOPort  Side=Left
  B : PMIOPort  Port=2  Side=Left
  C : PMIOPort  Port=3  Side=Left
  wires:
  Tm/1 -> ASM 575V 5000MVA Pm=4000 MW/1
  3500 MW/1 -> Terminator_1/1
  ASM 575V 5000MVA Pm=4000 MW/1 -> Terminator_2/1
  connections:
  A/RConn1 -- 22 000 MVA 735 kV/230 kV/LConn1
  B/RConn1 -- 22 000 MVA 735 kV/230 kV/LConn2
  C/RConn1 -- 22 000 MVA 735 kV/230 kV/LConn3
  230 kV/25 kV 18 000 MVA/LConn1 -- Load Flow Bus/LConn1 -- 22 000 MVA 735 kV/230 kV/RConn1 -- MTL 3000 Mvar/LConn1
  230 kV/25 kV 18 000 MVA/LConn2 -- 22 000 MVA 735 kV/230 kV/RConn2 -- MTL 3000 Mvar/LConn2
  230 kV/25 kV 18 000 MVA/LConn3 -- 22 000 MVA 735 kV/230 kV/RConn3 -- MTL 3000 Mvar/LConn3
  MTL 4000 MW1/LConn1 -- Load Flow Bus1/LConn1 -- MTL 4000 MW/LConn1 -- 230 kV/25 kV 18 000 MVA/RConn1 -- 3500 MW/LConn1 -- ASM 575V 5000MVA Pm=4000 MW/LConn1 -- 1.2  Mvar/LConn1
  MTL 4000 MW1/LConn2 -- MTL 4000 MW/LConn2 -- 230 kV/25 kV 18 000 MVA/RConn2 -- 3500 MW/LConn2 -- ASM 575V 5000MVA Pm=4000 MW/LConn2 -- 1.2  Mvar/LConn2
  230 kV/25 kV 18 000 MVA/RConn3 -- ASM 575V 5000MVA Pm=4000 MW/LConn3 -- 1.2  Mvar/LConn3 -- MTL 4000 MW1/LConn3 -- MTL 4000 MW/LConn3 -- 3500 MW/LConn3
